simulink model "negator"  (R2018a)
settings: Solver=VariableStepAuto  StartTime=0.0  StopTime=10.0  RelTol=1e-3
settings Model: Creator=Edoardo Debenedetti  LastModifiedBy=Edoardo Debenedetti

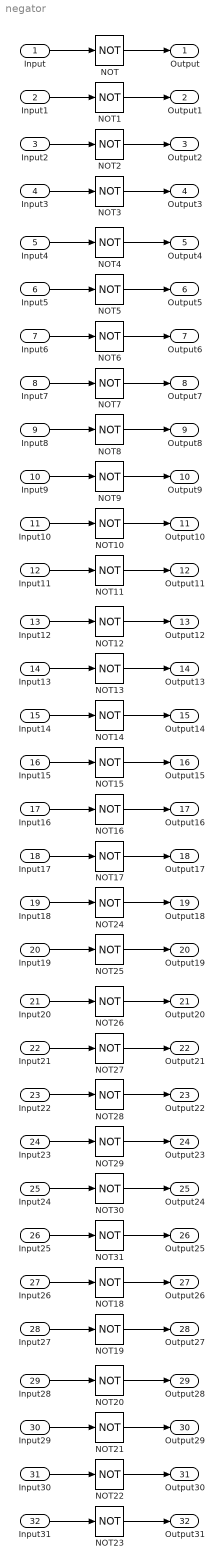
== system negator ==
  Input : Inport
  Input1 : Inport  Port=2
  Input2 : Inport  Port=3
  Input3 : Inport  Port=4
  Input4 : Inport  Port=5
  Input5 : Inport  Port=6
  Input6 : Inport  Port=7
  Input7 : Inport  Port=8
  Input8 : Inport  Port=9
  Input9 : Inport  Port=10
  Input10 : Inport  Port=11
  Input11 : Inport  Port=12
  Input12 : Inport  Port=13
  Input13 : Inport  Port=14
  Input14 : Inport  Port=15
  Input15 : Inport  Port=16
  Input16 : Inport  Port=17
  Input17 : Inport  Port=18
  Input18 : Inport  Port=19
  Input19 : Inport  Port=20
  Input20 : Inport  Port=21
  Input21 : Inport  Port=22
  Input22 : Inport  Port=23
  Input23 : Inport  Port=24
  Input24 : Inport  Port=25
  Input25 : Inport  Port=26
  Input26 : Inport  Port=27
  Input27 : Inport  Port=28
  Input28 : Inport  Port=29
  Input29 : Inport  Port=30
  Input30 : Inport  Port=31
  Input31 : Inport  Port=32
  NOT{,1..31} (32 alike) : Logic  Operator=NOT  IconShape=distinctive  AllPortsSameDT=off  OutDataTypeStr=boolean
  Output : Outport
  Output1 : Outport  Port=2
  Output2 : Outport  Port=3
  Output3 : Outport  Port=4
  Output4 : Outport  Port=5
  Output5 : Outport  Port=6
  Output6 : Outport  Port=7
  Output7 : Outport  Port=8
  Output8 : Outport  Port=9
  Output9 : Outport  Port=10
  Output10 : Outport  Port=11
  Output11 : Outport  Port=12
  Output12 : Outport  Port=13
  Output13 : Outport  Port=14
  Output14 : Outport  Port=15
  Output15 : Outport  Port=16
  Output16 : Outport  Port=17
  Output17 : Outport  Port=18
  Output18 : Outport  Port=19
  Output19 : Outport  Port=20
  Output20 : Outport  Port=21
  Output21 : Outport  Port=22
  Output22 : Outport  Port=23
  Output23 : Outport  Port=24
  Output24 : Outport  Port=25
  Output25 : Outport  Port=26
  Output26 : Outport  Port=27
  Output27 : Outport  Port=28
  Output28 : Outport  Port=29
  Output29 : Outport  Port=30
  Output30 : Outport  Port=31
  Output31 : Outport  Port=32
  wires:
  Input/1 -> NOT/1
  NOT/1 -> Output/1
  NOT1/1 -> Output1/1
  Input1/1 -> NOT1/1
  Input3/1 -> NOT3/1
  NOT3/1 -> Output3/1
  NOT2/1 -> Output2/1
  Input2/1 -> NOT2/1
  Input6/1 -> NOT6/1
  NOT6/1 -> Output6/1
  NOT7/1 -> Output7/1
  Input7/1 -> NOT7/1
  Input5/1 -> NOT5/1
  NOT5/1 -> Output5/1
  NOT4/1 -> Output4/1
  Input4/1 -> NOT4/1
  Input12/1 -> NOT12/1
  NOT12/1 -> Output12/1
  NOT13/1 -> Output13/1
  Input13/1 -> NOT13/1
  Input15/1 -> NOT15/1
  NOT15/1 -> Output15/1
  NOT14/1 -> Output14/1
  Input14/1 -> NOT14/1
  Input10/1 -> NOT10/1
  NOT10/1 -> Output10/1
  NOT11/1 -> Output11/1
  Input11/1 -> NOT11/1
  Input9/1 -> NOT9/1
  NOT9/1 -> Output9/1
  NOT8/1 -> Output8/1
  Input8/1 -> NOT8/1
  Input24/1 -> NOT30/1
  NOT30/1 -> Output24/1
  NOT31/1 -> Output25/1
  Input25/1 -> NOT31/1
  Input27/1 -> NOT19/1
  NOT19/1 -> Output27/1
  NOT18/1 -> Output26/1
  Input26/1 -> NOT18/1
  Input30/1 -> NOT22/1
  NOT22/1 -> Output30/1
  NOT23/1 -> Output31/1
  Input31/1 -> NOT23/1
  Input29/1 -> NOT21/1
  NOT21/1 -> Output29/1
  NOT20/1 -> Output28/1
  Input28/1 -> NOT20/1
  Input20/1 -> NOT26/1
  NOT26/1 -> Output20/1
  NOT27/1 -> Output21/1
  Input21/1 -> NOT27/1
  Input23/1 -> NOT29/1
  NOT29/1 -> Output23/1
  NOT28/1 -> Output22/1
  Input22/1 -> NOT28/1
  Input18/1 -> NOT24/1
  NOT24/1 -> Output18/1
  NOT25/1 -> Output19/1
  Input19/1 -> NOT25/1
  Input17/1 -> NOT17/1
  NOT17/1 -> Output17/1
  NOT16/1 -> Output16/1
  Input16/1 -> NOT16/1
